simulink model "Sistema"  (R2023a)
settings: Solver=ode15s  StartTime=0.0  StopTime=10.0  MaxStep=1E-3  RelTol=1e-3
libraries: fl_lib x14, nesl_utility x6, slpidlib x1
settings Model: Creator=lunit  LastModifiedBy=Dino
settings DataIOCC: SaveFormat=Array  ReturnWorkspaceOutputs=off  TimeSaveName=t
settings DebuggingCC: AlgebraicLoopMsg=none  ArtificialAlgebraicLoopMsg=none  MaxConsecutiveZCsMsg=none  UnconnectedInputMsg=warning  UnconnectedOutputMsg=warning  UnconnectedLineMsg=warning  ModelReferenceExtraNoncontSigs=none  OperatingPointInterfaceChecksumMismatchMsg=none
settings ModelReferenceCC: EnableRefExpFcnMdlSchedulingChecks=on
settings RTWCC: DLArmComputeVersion=19.05

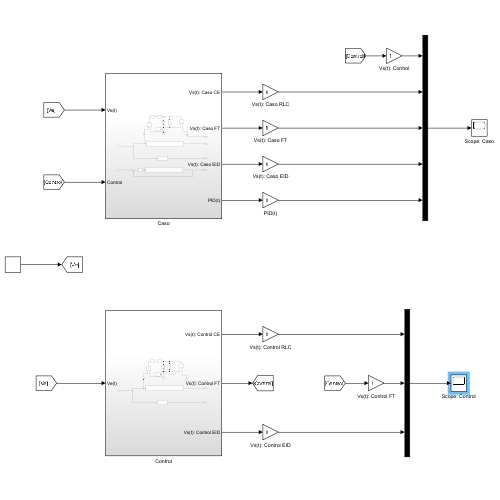
[thumbnail: Simulink's stored preview of the top-level diagram]
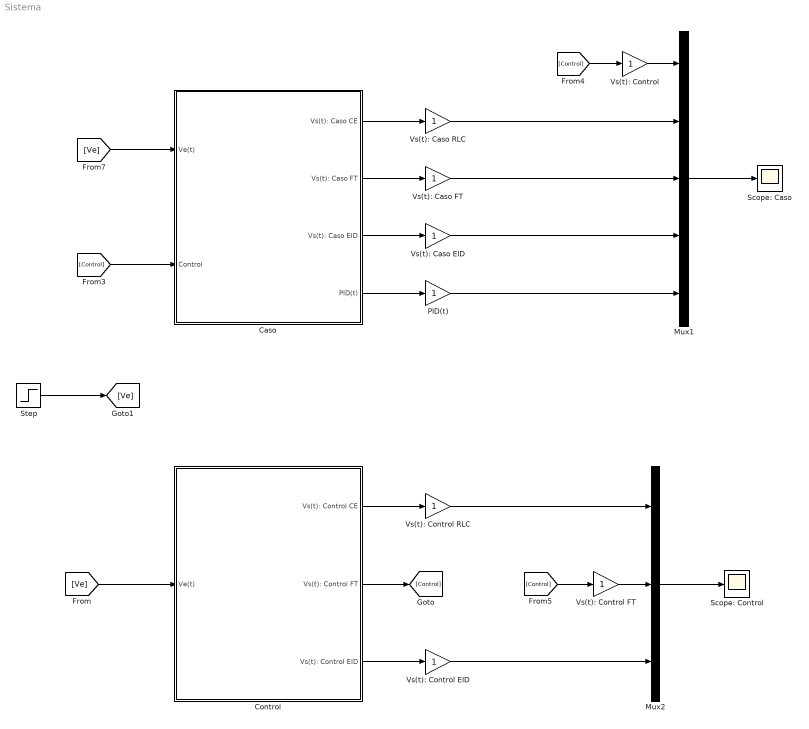
== system Sistema ==
  Caso : Subsystem
  Control : Subsystem
  Mux1 : Mux  Inputs=5
  Mux2 : Mux  Inputs=3
  PID(t) : Gain
  Scope: Caso : Scope
  Scope: Control : Scope
  Step : Step  SampleTime=0
  Vs(t): Caso EID : Gain
  Vs(t): Caso FT : Gain
  Vs(t): Caso RLC : Gain
  Vs(t): Control : Gain
  Vs(t): Control EID : Gain
  Vs(t): Control FT : Gain
  Vs(t): Control RLC : Gain
  wires:
  Mux1/1 -> Scope: Caso/1
  Caso/2(Vs(t): Caso FT) -> Vs(t): Caso FT/1
  PID(t)/1 -> Mux1/5
  Vs(t): Caso EID/1 -> Mux1/4
  Caso/4(PID(t)) -> PID(t)/1
  Vs(t): Caso FT/1 -> Mux1/3
  [Control] -> Caso/2(Control)
  Caso/3(Vs(t): Caso EID) -> Vs(t): Caso EID/1
  Caso/1(Vs(t): Caso CE) -> Vs(t): Caso RLC/1
  Vs(t): Caso RLC/1 -> Mux1/2
  Vs(t): Control EID/1 -> Mux2/3
  Mux2/1 -> Scope: Control/1
  Vs(t): Control RLC/1 -> Mux2/1
  [Ve] -> Caso/1(Ve(t))
  Step/1 -> [Ve]
  Vs(t): Control FT/1 -> Mux2/2
  [Control] -> Vs(t): Control FT/1
  Vs(t): Control/1 -> Mux1/1
  [Control] -> Vs(t): Control/1
  Control/1(Vs(t): Control CE) -> Vs(t): Control RLC/1
  Control/2(Vs(t): Control FT) -> [Control]
  Control/3(Vs(t): Control EID) -> Vs(t): Control EID/1
  [Ve] -> Control/1(Ve(t))

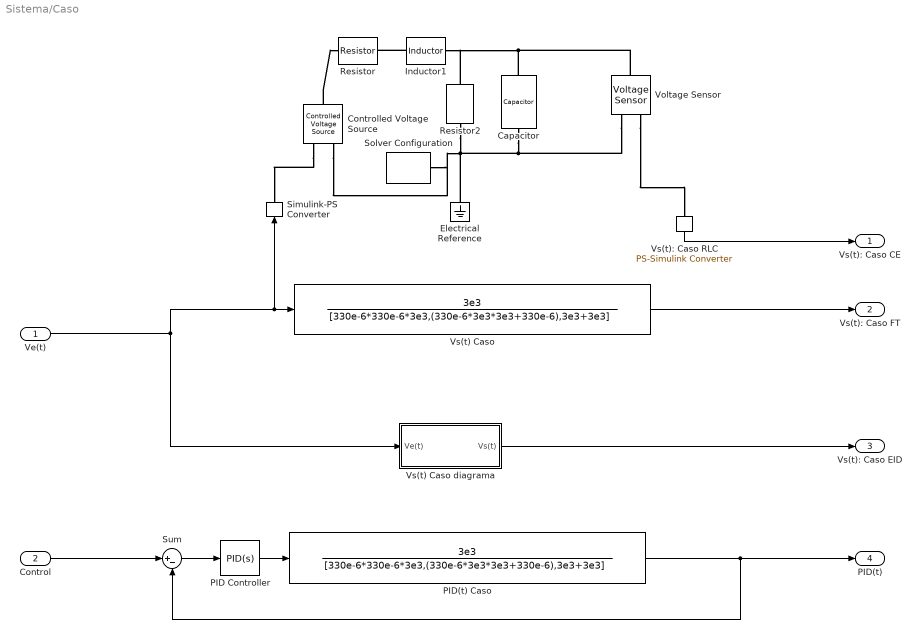
== system Sistema/Caso ==
  Ve(t) : Inport
  Control : Inport  Port=2
  Capacitor : fl_lib/Electrical/Electrical Elements/Capacitor  c=330 uF  r=1e-6 Ohm  g=0 1/Ohm  i_specify=off  i_priority=None  i=0 A  i_nominal_specify=off  i_nominal_unit=A  i_nominal_value=1  v_specify=off  v_priority=None  v=0 V  v_nominal_specify=off  v_nominal_unit=V  v_nominal_value=1  vc_specify=off  vc_priority=High  vc=0 V  vc_nominal_specify=off  vc_nominal_unit=V  vc_nominal_value=1
  Controlled Voltage Source : fl_lib/Electrical/Electrical Sources/Controlled Voltage Source
  Electrical Reference : fl_lib/Electrical/Electrical Elements/Electrical Reference
  Inductor1 : fl_lib/Electrical/Electrical Elements/Inductor  l=330 uH  r=0 Ohm  g=1e-9 1/Ohm  i_specify=off  i_priority=None  i=0 A  i_nominal_specify=off  i_nominal_unit=A  i_nominal_value=1  v_specify=off  v_priority=None  v=0 V  v_nominal_specify=off  v_nominal_unit=V  v_nominal_value=1  i_L_specify=off  i_L_priority=High  i_L=0 A  i_L_nominal_specify=off  i_L_nominal_unit=A  i_L_nominal_value=1
  PID Controller : slpidlib/PID Controller  Controller=PID  Form=Parallel  TimeDomain=Continuous-time  UseExternalTs=off  SampleTime=-1  IntegratorMethod=Forward Euler  FilterMethod=Forward Euler  ControllerParametersSource=internal  P=31.6345631855362  I=282.224740454676  UseKiTs=off  D=0.224972715483495  N=60.9899542534147  UseFilter=on  TunerSelectOption=Transfer Function Based (PID Tuner App)  InitialConditionSource=internal  InitialConditionForIntegrator=0  InitialConditionForFilter=0  DifferentiatorICPrevScaledInput=0  ExternalReset=none  TrackingMode=off  Kt=1  LimitOutput=off  SatLimitsSource=internal  UpperSaturationLimit=inf  LowerSaturationLimit=-inf  LinearizeAsGain=on  AntiWindupMode=none  Kb=1  LimitIntegrator=off  UpperIntegratorSaturationLimit=inf  LowerIntegratorSaturationLimit=-inf  POutMin=[]  POutMax=[]  IOutMin=[]  IOutMax=[]  DOutMin=[]  DOutMax=[]  NOutMin=[]  NOutMax=[]  SumOutMin=[]  SumOutMax=[]  SaturationOutMin=[]  SaturationOutMax=[]  PParamMin=[]  PParamMax=[]  IParamMin=[]  IParamMax=[]  DParamMin=[]  DParamMax=[]  NParamMin=[]  NParamMax=[]  KbParamMin=[]  KbParamMax=[]  KtParamMin=[]  KtParamMax=[]  KbOutMin=[]  KbOutMax=[]  KtOutMin=[]  KtOutMax=[]  IntegratorOutMin=[]  IntegratorOutMax=[]  FilterOutMin=[]  FilterOutMax=[]  SumI1OutMin=[]  SumI1OutMax=[]  SumI2OutMin=[]  SumI2OutMax=[]  SumI3OutMin=[]  SumI3OutMax=[]  SumI4OutMin=[]  SumI4OutMax=[]  SumDOutMin=[]  SumDOutMax=[]  DifferentiatorOutMin=[]  DifferentiatorOutMax=[]  FilterDiffOutCoefMin=[]  FilterDiffOutCoefMax=[]  ReciprocalOutMin=[]  ReciprocalOutMax=[]  SumDenOutMin=[]  SumDenOutMax=[]  SumNumOutMin=[]  SumNumOutMax=[]  DivideOutMin=[]  DivideOutMax=[]  UdiffTsProdOutMin=[]  UdiffTsProdOutMax=[]  NTsProdOutMin=[]  NTsProdOutMax=[]  UintegralTsProdOutMin=[]  UintegralTsProdOutMax=[]  UngainTsProdOutMin=[]  UngainTsProdOutMax=[]  ClampingZeroOutDataTypeStr=Inherit: Inherit via back propagation  ClampingZeroOutMin=[]  ClampingZeroOutMax=[]  FilterDenConstantOutDataTypeStr=Inherit: Inherit via back propagation  FilterDenConstantOutMin=[]  FilterDenConstantOutMax=[]  PCopyOutDataTypeStr=Inherit: Inherit via back propagation  PCopyOutMin=[]  PCopyOutMax=[]  NCopyOutDataTypeStr=Inherit: Inherit via back propagation  NCopyOutMin=[]  NCopyOutMax=[]  IntegratorContinuousStateAttributes=''  IntegratorStateMustResolveToSignalObject=off  IntegratorRTWStateStorageClass=Auto  FilterContinuousStateAttributes=''  FilterStateMustResolveToSignalObject=off  FilterRTWStateStorageClass=Auto  ParallelPVariant=InternalParameters  IdealPVariant=Disabled  IVariant=InternalParameters  DVariant=InternalParameters  IntegratorVariant=Continuous  SatVariant=Disabled  AWVariant=Passthrough  PCopyVariant=Disabled  TRVariant=Disabled  FdbkBlocksVariant=Forward  IdealPFdbkVariant=Disabled  SatFdbkVariant=Disabled  DerivativeFilterVariant=ContFilter  NVariant=InternalParameters  NCopyVariant=Disabled  FilterICVariant=InternalICsFilter  IntegratorICVariant=InternalICs  ExternalResetVariant=Disabled  TRSumVariant=Passthrough  SumFdbkVariant=Disabled  SumVariant=Sum_PID  TsampFilterVariant=InternalTs  TsampNgainVariant=Passthrough  TsampIntegralVariant=Disabled_SignalSpec  ExternalSaturationOutDataTypeStr=Inherit: Same as second input
  PID(t) Caso : TransferFcn  Numerator=3e3  Denominator=[330e-6*330e-6*3e3,(330e-6*3e3*3e3+330e-6),3e3+3e3]
  Resistor : fl_lib/Electrical/Electrical Elements/Resistor  R=3 kOhm  i_specify=off  i_priority=None  i=0 A  i_nominal_specify=off  i_nominal_unit=A  i_nominal_value=1  v_specify=off  v_priority=None  v=0 V  v_nominal_specify=off  v_nominal_unit=V  v_nominal_value=1
  Resistor2 : fl_lib/Electrical/Electrical Elements/Resistor  R=3 kOhm  i_specify=off  i_priority=None  i=0 A  i_nominal_specify=off  i_nominal_unit=A  i_nominal_value=1  v_specify=off  v_priority=None  v=0 V  v_nominal_specify=off  v_nominal_unit=V  v_nominal_value=1
  Simulink-PS Converter : nesl_utility/Simulink-PS Converter  PhysicalDomain=network_engine_domain  SubClassName=ps_input  LeftPortType=input  RightPortType=output  PseudoPeriodic=off  Frequencies=[]  NoiseDistribution=none  NoiseParameters=[]  Unit=1  AffineConversion=off  FilteringAndDerivatives=provide  SimscapeFilterOrder=1  InputFilterTimeConstant=0.001  UdotUserProvided=0
  Solver Configuration : nesl_utility/Solver Configuration  PhysicalDomain=network_engine_domain  SubClassName=solver  LeftPortType=input  RightPortType=generic  Tones=[]  Harmonics=[]  SimulateNoise=off  Profile=off  UseLocalSampling=off  EnableSwitchedLinearOptims=on  FrequencyDomain=off  UseCCode=off  RelTol=0.001  AbsTol=0.001  MinStep=1e-09  ToWorkspace=off  RevertToSquareIcSolve=off  NumHomotopyIterations=100  PhasorMode=off  PhasorModeNumHarmonics=1  ConsistencySolver=NEWTON_XTOL_AFTER_FTOL  IndexReductionMethod=DerivativeReplacement  DoDC=off  ResidualTolerance=1e-09  ConsistencyTolSource=GLOBAL  ConsistencyAbsTol=0.001  ConsistencyRelTol=0.001  ConsistencyTolFactor=0.001  UseLocalSolver=off  LocalSolverChoice=NE_BACKWARD_EULER_ADVANCER  ResolveIndetEquations=on  FunctionEvalNumThread=1  LocalSolverSampleTime=0.001  DoFixedCost=off  MaxNonlinIter=3  MaxModeIter=2  ComputeImpulses=off  ImpulseIterations=2  LinearAlgebra=auto  LinearAlgebraNumThread=0  EquationFormulation=NE_TIME_EF  DelaysMemoryBudget=1024  AutomaticFiltering=on  FilteringTimeConstant=0.001  PartitionStorageMethod=AS_NEEDED  PartitionMemoryBudget=1024  PartitionMethod=ROBUST
  Sum : Sum  Inputs=|+-
  Voltage Sensor : fl_lib/Electrical/Electrical Sensors/Voltage Sensor
  Vs(t) Caso : TransferFcn  Numerator=3e3  Denominator=[330e-6*330e-6*3e3,(330e-6*3e3*3e3+330e-6),3e3+3e3]
  Vs(t) Caso diagrama : Subsystem
  Vs(t): Caso RLC : nesl_utility/PS-Simulink Converter  PhysicalDomain=network_engine_domain  SubClassName=ps_output  LeftPortType=input  RightPortType=output  PseudoPeriodic=off  Frequencies=[]  VectorFormat=1-D array  Unit=inherit  AffineConversion=off
  Vs(t): Caso CE : Outport
  Vs(t): Caso FT : Outport  Port=2
  Vs(t): Caso EID : Outport  Port=3
  PID(t) : Outport  Port=4
  wires:
  Vs(t) Caso/1 -> Vs(t): Caso FT/1
  Ve(t)/1 -> Vs(t) Caso diagrama/1(Ve(t)), Simulink-PS Converter/1, Vs(t) Caso/1
  Vs(t): Caso RLC/1 -> Vs(t): Caso CE/1
  Vs(t) Caso diagrama/1(Vs(t)) -> Vs(t): Caso EID/1
  Control/1 -> Sum/1
  PID Controller/1 -> PID(t) Caso/1
  Sum/1 -> PID Controller/1
  PID(t) Caso/1 -> PID(t)/1, Sum/2
  connections:
  Controlled Voltage Source/LConn1 -- Resistor/LConn1
  Voltage Sensor/LConn1 -- Resistor2/LConn1 -- Inductor1/RConn1 -- Capacitor/LConn1
  Controlled Voltage Source/RConn1 -- Simulink-PS Converter/RConn1
  Voltage Sensor/RConn1 -- Vs(t): Caso RLC/LConn1
  Voltage Sensor/RConn2 -- Capacitor/RConn1 -- Resistor2/RConn1 -- Controlled Voltage Source/RConn2 -- Solver Configuration/RConn1 -- Electrical Reference/LConn1
  Inductor1/LConn1 -- Resistor/RConn1

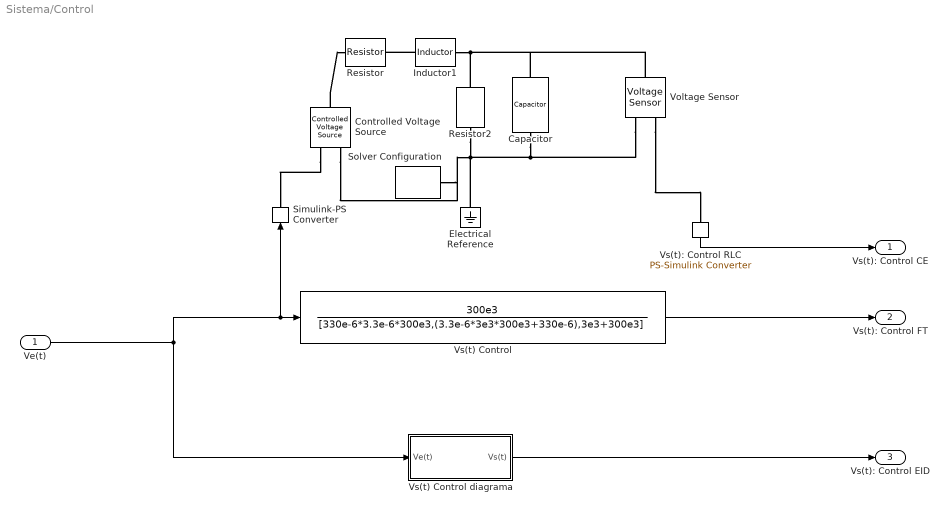
== system Sistema/Control ==
  Ve(t) : Inport
  Capacitor : fl_lib/Electrical/Electrical Elements/Capacitor  c=3.3 uF  r=1e-6 Ohm  g=0 1/Ohm  i_specify=off  i_priority=None  i=0 A  i_nominal_specify=off  i_nominal_unit=A  i_nominal_value=1  v_specify=off  v_priority=None  v=0 V  v_nominal_specify=off  v_nominal_unit=V  v_nominal_value=1  vc_specify=off  vc_priority=High  vc=0 V  vc_nominal_specify=off  vc_nominal_unit=V  vc_nominal_value=1
  Controlled Voltage Source : fl_lib/Electrical/Electrical Sources/Controlled Voltage Source
  Electrical Reference : fl_lib/Electrical/Electrical Elements/Electrical Reference
  Inductor1 : fl_lib/Electrical/Electrical Elements/Inductor  l=330 uH  r=0 Ohm  g=1e-9 1/Ohm  i_specify=off  i_priority=None  i=0 A  i_nominal_specify=off  i_nominal_unit=A  i_nominal_value=1  v_specify=off  v_priority=None  v=0 V  v_nominal_specify=off  v_nominal_unit=V  v_nominal_value=1  i_L_specify=off  i_L_priority=High  i_L=0 A  i_L_nominal_specify=off  i_L_nominal_unit=A  i_L_nominal_value=1
  Resistor : fl_lib/Electrical/Electrical Elements/Resistor  R=3 kOhm  i_specify=off  i_priority=None  i=0 A  i_nominal_specify=off  i_nominal_unit=A  i_nominal_value=1  v_specify=off  v_priority=None  v=0 V  v_nominal_specify=off  v_nominal_unit=V  v_nominal_value=1
  Resistor2 : fl_lib/Electrical/Electrical Elements/Resistor  R=300 kOhm  i_specify=off  i_priority=None  i=0 A  i_nominal_specify=off  i_nominal_unit=A  i_nominal_value=1  v_specify=off  v_priority=None  v=0 V  v_nominal_specify=off  v_nominal_unit=V  v_nominal_value=1
  Simulink-PS Converter : nesl_utility/Simulink-PS Converter  PhysicalDomain=network_engine_domain  SubClassName=ps_input  LeftPortType=input  RightPortType=output  PseudoPeriodic=off  Frequencies=[]  NoiseDistribution=none  NoiseParameters=[]  Unit=1  AffineConversion=off  FilteringAndDerivatives=provide  SimscapeFilterOrder=1  InputFilterTimeConstant=0.001  UdotUserProvided=0
  Solver Configuration : nesl_utility/Solver Configuration  PhysicalDomain=network_engine_domain  SubClassName=solver  LeftPortType=input  RightPortType=generic  Tones=[]  Harmonics=[]  SimulateNoise=off  Profile=off  UseLocalSampling=off  EnableSwitchedLinearOptims=on  FrequencyDomain=off  UseCCode=off  RelTol=0.001  AbsTol=0.001  MinStep=1e-09  ToWorkspace=off  RevertToSquareIcSolve=off  NumHomotopyIterations=100  PhasorMode=off  PhasorModeNumHarmonics=1  ConsistencySolver=NEWTON_XTOL_AFTER_FTOL  IndexReductionMethod=DerivativeReplacement  DoDC=off  ResidualTolerance=1e-09  ConsistencyTolSource=GLOBAL  ConsistencyAbsTol=0.001  ConsistencyRelTol=0.001  ConsistencyTolFactor=0.001  UseLocalSolver=off  LocalSolverChoice=NE_BACKWARD_EULER_ADVANCER  ResolveIndetEquations=on  FunctionEvalNumThread=1  LocalSolverSampleTime=0.001  DoFixedCost=off  MaxNonlinIter=3  MaxModeIter=2  ComputeImpulses=off  ImpulseIterations=2  LinearAlgebra=auto  LinearAlgebraNumThread=0  EquationFormulation=NE_TIME_EF  DelaysMemoryBudget=1024  AutomaticFiltering=on  FilteringTimeConstant=0.001  PartitionStorageMethod=AS_NEEDED  PartitionMemoryBudget=1024  PartitionMethod=ROBUST
  Voltage Sensor : fl_lib/Electrical/Electrical Sensors/Voltage Sensor
  Vs(t) Control : TransferFcn  Numerator=300e3  Denominator=[330e-6*3.3e-6*300e3,(3.3e-6*3e3*300e3+330e-6),3e3+300e3]
  Vs(t) Control diagrama : Subsystem
  Vs(t): Control RLC : nesl_utility/PS-Simulink Converter  PhysicalDomain=network_engine_domain  SubClassName=ps_output  LeftPortType=input  RightPortType=output  PseudoPeriodic=off  Frequencies=[]  VectorFormat=1-D array  Unit=inherit  AffineConversion=off
  Vs(t): Control CE : Outport
  Vs(t): Control FT : Outport  Port=2
  Vs(t): Control EID : Outport  Port=3
  wires:
  Vs(t) Control diagrama/1(Vs(t)) -> Vs(t): Control EID/1
  Vs(t) Control/1 -> Vs(t): Control FT/1
  Ve(t)/1 -> Vs(t) Control diagrama/1(Ve(t)), Simulink-PS Converter/1, Vs(t) Control/1
  Vs(t): Control RLC/1 -> Vs(t): Control CE/1
  connections:
  Voltage Sensor/RConn2 -- Capacitor/RConn1 -- Resistor2/RConn1 -- Controlled Voltage Source/RConn2 -- Solver Configuration/RConn1 -- Electrical Reference/LConn1
  Inductor1/RConn1 -- Capacitor/LConn1 -- Voltage Sensor/LConn1 -- Resistor2/LConn1
  Inductor1/LConn1 -- Resistor/RConn1
  Voltage Sensor/RConn1 -- Vs(t): Control RLC/LConn1
  Controlled Voltage Source/RConn1 -- Simulink-PS Converter/RConn1
  Controlled Voltage Source/LConn1 -- Resistor/LConn1

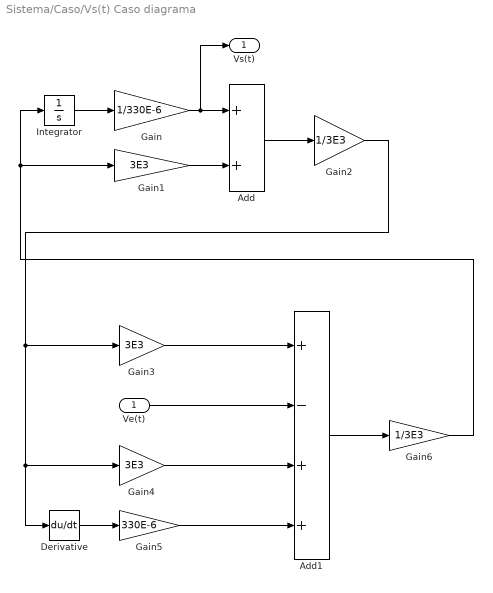
== system Sistema/Caso/Vs(t) Caso diagrama ==
  Ve(t) : Inport
  Add : Sum
  Add1 : Sum  Inputs=+-++
  Derivative : Derivative
  Gain : Gain  Gain=1/330E-6
  Gain1 : Gain  Gain=3E3
  Gain2 : Gain  Gain=1/3E3
  Gain3 : Gain  Gain=3E3
  Gain4 : Gain  Gain=3E3
  Gain5 : Gain  Gain=330E-6
  Gain6 : Gain  Gain=1/3E3
  Integrator : Integrator
  Vs(t) : Outport
  wires:
  Gain1/1 -> Add/2
  Gain/1 -> Vs(t)/1, Add/1
  Add/1 -> Gain2/1
  Derivative/1 -> Gain5/1
  Integrator/1 -> Gain/1
  Gain3/1 -> Add1/1
  Ve(t)/1 -> Add1/2
  Gain4/1 -> Add1/3
  Gain5/1 -> Add1/4
  Add1/1 -> Gain6/1
  Gain2/1 -> Gain3/1, Gain4/1, Derivative/1
  Gain6/1 -> Gain1/1, Integrator/1

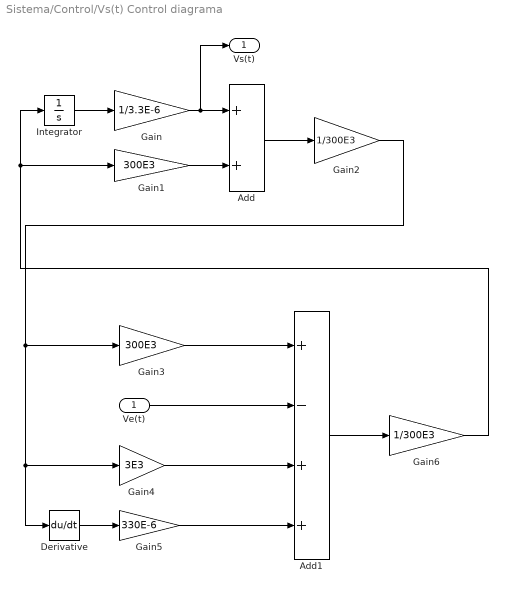
== system Sistema/Control/Vs(t) Control diagrama ==
  Ve(t) : Inport
  Add : Sum
  Add1 : Sum  Inputs=+-++
  Derivative : Derivative
  Gain : Gain  Gain=1/3.3E-6
  Gain1 : Gain  Gain=300E3
  Gain2 : Gain  Gain=1/300E3
  Gain3 : Gain  Gain=300E3
  Gain4 : Gain  Gain=3E3
  Gain5 : Gain  Gain=330E-6
  Gain6 : Gain  Gain=1/300E3
  Integrator : Integrator
  Vs(t) : Outport
  wires:
  Gain1/1 -> Add/2
  Gain/1 -> Vs(t)/1, Add/1
  Add/1 -> Gain2/1
  Derivative/1 -> Gain5/1
  Integrator/1 -> Gain/1
  Gain3/1 -> Add1/1
  Ve(t)/1 -> Add1/2
  Gain4/1 -> Add1/3
  Gain5/1 -> Add1/4
  Add1/1 -> Gain6/1
  Gain2/1 -> Gain3/1, Gain4/1, Derivative/1
  Gain6/1 -> Gain1/1, Integrator/1
